simulink model "penduloDobleVersionFinal"  (R2021a)
settings: Solver=ode4  StartTime=0.0  StopTime=25  FixedStep=1e-3  RelTol=1e-3
PreLoadFcn:
  | cuentas_pendulo_doble_final;
InitFcn:
  | cuentas_pendulo_doble_final;
values from neighbouring files (symbols this model uses):
  I0 = 0    [TPF_Control_Automatico.m]    (also in cuentas_pendulo_doble_final.m)
  I1 = m1_value*(((L1_value)^2)/12)    (= 0.0833333333333)    [TPF_Control_Automatico.m]    (also in cuentas_pendulo_doble_final.m; cuentas_prueba.m = 0.0104166666667)
  I2 = m2_value*(((L2_value)^2)/12)    (= 0.1875)    [TPF_Control_Automatico.m]    (also in cuentas_pendulo_doble_final.m; cuentas_prueba.m = 0.03515625)
  K = place(sys.A, sys.B, [-3 -2.5 -2.4 -2 -1.9 -1.8])    [TPF_Control_Automatico.m]    (also in cuentas_pendulo_doble.m = acker(A,B,[0.002,-0.001,-0.001,-0.001,-0.001,-0.001]); cuentas_pendulo_doble_final.m = place(sys.A, sys.B, [-4 -3.5 -3 -2.5 -2 -1.5]); cuentas_prueba.m = acker(sys.A, sys.B, [-3 -3 -2 -2]))
  Ka = Ka(1:6)    [cuentas_pendulo_doble_final.m]    (also in cuentas_prueba.m = Ka(1:4))
  KaDisc = KDisc2(1:6)    [cuentas_pendulo_doble_final.m]    (also in cuentas_prueba.m = KDisc2(1:4))
  Kai = Ka(7)    [cuentas_pendulo_doble_final.m]    (also in cuentas_prueba.m = Ka(5))
  KaiDisc = KDisc2(7)    [cuentas_pendulo_doble_final.m]    (also in cuentas_prueba.m = KDisc2(5))
  KDisc = place(sysDisc.A, sysDisc.B, exp([-1.5 -1.6 -1.7 -2 -2.1 -2.2].*Ts))    [TPF_Control_Automatico.m]    (also in cuentas_pendulo_doble_final.m = place(sysDisc.A, sysDisc.B, exp([-3.5 -3 -2.5 -2 -1.5 -1].*T; cuentas_prueba.m = acker(sysDisc.A, sysDisc.B, exp([-2 -2 -1 -1].*Ts)))
  L = place((sys.A)',(sys.C)', [-3 -2.5 -2.4 -2 -1.9 -1.8].*10)'    [TPF_Control_Automatico.m]    (also in cuentas_pendulo_doble.m = [zeros(3,1); cuentas_pendulo_doble_final.m = place((sys.A)',(sys.C)', [-4 -3.5 -3 -2.5 -2 -1.5].*15)'; cuentas_prueba.m = place((sys.A)',(sys.C)', [-25 -20 -35 -30])')
  L1_value = 1    [TPF_Control_Automatico.m]    (also in cuentas_pendulo_doble.m = 0.5; cuentas_pendulo_doble_final.m; cuentas_prueba.m = 0.5)
  L2_value = 1.5    [TPF_Control_Automatico.m]    (also in cuentas_pendulo_doble.m = 0.75; cuentas_pendulo_doble_final.m; cuentas_prueba.m = 0.75)
  LDisc = place((sysDisc.A)',(sysDisc.C)', exp(([-1.5 -1.6 -1.7 -2 -2.1 -2.2].*20).*Ts))'    [TPF_Control_Automatico.m]    (also in cuentas_pendulo_doble_final.m = place((sysDisc.A)',(sysDisc.C)', exp(([-3.5 -3 -2.5 -2 -1.5 ; cuentas_prueba.m = place((sysDisc.A)',(sysDisc.C)', exp([-20 -15 -25 -30].*Ts)))
  m0_value = 5    [TPF_Control_Automatico.m]    (also in cuentas_pendulo_doble.m = 1.5; cuentas_pendulo_doble_final.m; cuentas_prueba.m = 1.5)
  m1_value = 1    [TPF_Control_Automatico.m]    (also in cuentas_pendulo_doble.m = 0.5; cuentas_pendulo_doble_final.m; cuentas_prueba.m = 0.5)
  m2_value = 1    [TPF_Control_Automatico.m]    (also in cuentas_pendulo_doble.m = 0.75; cuentas_pendulo_doble_final.m; cuentas_prueba.m = 0.75)
  s = tf('s')    [TPF_Control_Automatico.m]    (also in cuentas_pendulo_doble.m; cuentas_pendulo_doble_final.m; cuentas_prueba.m)
  sys = ss(A,B,C,D)    [TPF_Control_Automatico.m]    (also in cuentas_pendulo_doble_final.m; cuentas_prueba.m)
  sysDisc = c2d(sys, Ts, 'tustin')    [TPF_Control_Automatico.m]    (also in cuentas_pendulo_doble_final.m; cuentas_prueba.m)
  Ts = 0.03    [TPF_Control_Automatico.m]    (also in cuentas_pendulo_doble_final.m = 0.025; cuentas_prueba.m = 0.1)
  Ts2 = 0.01    [cuentas_pendulo_doble_final.m]    (also in cuentas_prueba.m = 0.05)
undefined symbols (not defined in the file or in its folder): DiscIntNeverNeededParam, X, Y, Z
libraries: sm_lib x100, nesl_utility x40, eeGeneralControl x5
(part 4 of 4)

== system penduloDobleVersionFinal/Control por realimentacion con obs discreto/Planta/Base ==
  Base : sm_lib/Body Elements/Brick Solid  GraphicAmbientColor=[0.15 0.15 0.15 1.0]  BasedOnType=Mass  BrickDimensions=[20 1 0.01]  BrickDimensionUnits=m  CenterOfMass=[0 0 0]  CenterOfMassUnits=m  GraphicDiffuseColor=[0.7 0.7 0.7]  Density=1000  DensityUnits=kg/m^3  DoExposeReferenceFrame=on  GraphicEmissiveColor=[0.0 0.0 0.0 1.0]  ExportEntireGeometry=off  SerializedFrames=<Frames/>  MarkerShape=Sphere  MarkerSize=10  GraphicType=FromGeometry  InertiaType=CalculateFromGeometry  Mass=10  MassUnits=kg  MomentsOfInertia=[1 1 1]  MomentsOfInertiaUnits=kg*m^2  GraphicOpacity=1.0  ProductsOfInertia=[0 0 0]  ProductsOfInertiaUnits=kg*m^2  GraphicShininess=75  GraphicSpecularColor=[0.5 0.5 0.5 1.0]  GraphicVisPropType=SimpleVisualProperties
  Base1 : sm_lib/Body Elements/Brick Solid  GraphicAmbientColor=[0.15 0.15 0.15 1.0]  BasedOnType=Mass  BrickDimensions=[20 0.05 0.0805]  BrickDimensionUnits=m  CenterOfMass=[0 0 0]  CenterOfMassUnits=m  GraphicDiffuseColor=[0.6 0.6 0.6]  Density=1000  DensityUnits=kg/m^3  DoExposeReferenceFrame=off  GraphicEmissiveColor=[0.0 0.0 0.0 1.0]  ExportEntireGeometry=off  SerializedFrames=<Frames><Frame><Id>Frame1</Id><Value><Name>F1</Name><Origin><Source>GeometricFeature</Source><FeatureName>-y +z curve</FeatureName></Origin><PrimaryAxis><DefinedDirection>+Z</DefinedDirection><Source>ReferenceFrame</Source><SourceDirection>+Z</SourceDirection><FeatureName></FeatureName></PrimaryAxis><SecondaryAxis><DefinedDirection>+X</DefinedDirection><Source>ReferenceFrame</Source><SourceDirection>+X</SourceDirection><FeatureName></FeatureName></SecondaryAxis></Value></Frame></Frames>  MarkerShape=Sphere  MarkerSize=10  GraphicType=FromGeometry  InertiaType=CalculateFromGeometry  Mass=10  MassUnits=kg  MomentsOfInertia=[1 1 1]  MomentsOfInertiaUnits=kg*m^2  GraphicOpacity=1.0  ProductsOfInertia=[0 0 0]  ProductsOfInertiaUnits=kg*m^2  GraphicShininess=75  GraphicSpecularColor=[0.5 0.5 0.5 1.0]  GraphicVisPropType=SimpleVisualProperties
  Base2 : sm_lib/Body Elements/Brick Solid  GraphicAmbientColor=[0.15 0.15 0.15 1.0]  BasedOnType=Mass  BrickDimensions=[20 0.05 0.0805]  BrickDimensionUnits=m  CenterOfMass=[0 0 0]  CenterOfMassUnits=m  GraphicDiffuseColor=[0.6 0.6 0.6]  Density=1000  DensityUnits=kg/m^3  DoExposeReferenceFrame=off  GraphicEmissiveColor=[0.0 0.0 0.0 1.0]  ExportEntireGeometry=off  SerializedFrames=<Frames><Frame><Id>Frame1</Id><Value><Name>F1</Name><Origin><Source>GeometricFeature</Source><FeatureName>-y +z curve</FeatureName></Origin><PrimaryAxis><DefinedDirection>+Z</DefinedDirection><Source>ReferenceFrame</Source><SourceDirection>+Z</SourceDirection><FeatureName></FeatureName></PrimaryAxis><SecondaryAxis><DefinedDirection>+X</DefinedDirection><Source>ReferenceFrame</Source><SourceDirection>+X</SourceDirection><FeatureName></FeatureName></SecondaryAxis></Value></Frame></Frames>  MarkerShape=Sphere  MarkerSize=10  GraphicType=FromGeometry  InertiaType=CalculateFromGeometry  Mass=10  MassUnits=kg  MomentsOfInertia=[1 1 1]  MomentsOfInertiaUnits=kg*m^2  GraphicOpacity=1.0  ProductsOfInertia=[0 0 0]  ProductsOfInertiaUnits=kg*m^2  GraphicShininess=75  GraphicSpecularColor=[0.5 0.5 0.5 1.0]  GraphicVisPropType=SimpleVisualProperties
  T1 : sm_lib/Frames and Transforms/Rigid Transform  TranslationMethod=StandardAxis  TranslationStandardOffset=-0.0255  TranslationLengthUnit=m  TranslationStandardAxis=+Z  TranslationCartesianOffset=[0 0 0]  TranslationROffset=0  TranslationROffsetUnits=m  TranslationZOffset=0  TranslationZOffsetUnits=m  TranslationThetaOffset=0  TranslationThetaOffsetUnits=deg  RotationMethod=RotationSequence  RotationAngleUnits=deg  RotationStandardAxis=+Z  RotationAngle=0.0  RotationArbitraryAxis=[0 0 1]  FollAlignAxisA=+X  BaseAlignAxisA=+Y  FollAlignAxisB=+Y  BaseAlignAxisB=+Z  RotationSequenceAxes=FollowerAxes  RotationSequence=XYZ  RotationSequenceAngles=[0 0 0]  RotationSequenceAnglesUnits=deg  RotationMatrix=[1 0 0; 0 1 0; 0 0 1]
  T2 : sm_lib/Frames and Transforms/Rigid Transform  TranslationMethod=StandardAxis  TranslationStandardOffset=0.05  TranslationLengthUnit=m  TranslationStandardAxis=+Z  TranslationCartesianOffset=[0 0 0]  TranslationROffset=0  TranslationROffsetUnits=m  TranslationZOffset=0  TranslationZOffsetUnits=m  TranslationThetaOffset=0  TranslationThetaOffsetUnits=deg  RotationMethod=RotationSequence  RotationAngleUnits=deg  RotationStandardAxis=+Z  RotationAngle=0.0  RotationArbitraryAxis=[0 0 1]  FollAlignAxisA=+X  BaseAlignAxisA=+Y  FollAlignAxisB=+Y  BaseAlignAxisB=+Z  RotationSequenceAxes=FollowerAxes  RotationSequence=XYZ  RotationSequenceAngles=[0 0 0]  RotationSequenceAnglesUnits=deg  RotationMatrix=[1 0 0; 0 1 0; 0 0 1]
  T3 : sm_lib/Frames and Transforms/Rigid Transform  TranslationMethod=StandardAxis  TranslationStandardOffset=0.5  TranslationLengthUnit=m  TranslationStandardAxis=+Y  TranslationCartesianOffset=[0 0 0]  TranslationROffset=0  TranslationROffsetUnits=m  TranslationZOffset=0  TranslationZOffsetUnits=m  TranslationThetaOffset=0  TranslationThetaOffsetUnits=deg  RotationMethod=RotationSequence  RotationAngleUnits=deg  RotationStandardAxis=+Z  RotationAngle=0.0  RotationArbitraryAxis=[0 0 1]  FollAlignAxisA=+X  BaseAlignAxisA=+Y  FollAlignAxisB=+Y  BaseAlignAxisB=+Z  RotationSequenceAxes=FollowerAxes  RotationSequence=XYZ  RotationSequenceAngles=[0 0 0]  RotationSequenceAnglesUnits=deg  RotationMatrix=[1 0 0; 0 1 0; 0 0 1]
  T4 : sm_lib/Frames and Transforms/Rigid Transform  TranslationMethod=StandardAxis  TranslationStandardOffset=0.05  TranslationLengthUnit=m  TranslationStandardAxis=+Z  TranslationCartesianOffset=[0 0 0]  TranslationROffset=0  TranslationROffsetUnits=m  TranslationZOffset=0  TranslationZOffsetUnits=m  TranslationThetaOffset=0  TranslationThetaOffsetUnits=deg  RotationMethod=RotationSequence  RotationAngleUnits=deg  RotationStandardAxis=+Z  RotationAngle=0.0  RotationArbitraryAxis=[0 0 1]  FollAlignAxisA=+X  BaseAlignAxisA=+Y  FollAlignAxisB=+Y  BaseAlignAxisB=+Z  RotationSequenceAxes=FollowerAxes  RotationSequence=XYZ  RotationSequenceAngles=[0 0 0]  RotationSequenceAnglesUnits=deg  RotationMatrix=[1 0 0; 0 1 0; 0 0 1]
  T5 : sm_lib/Frames and Transforms/Rigid Transform  TranslationMethod=StandardAxis  TranslationStandardOffset=0.55  TranslationLengthUnit=m  TranslationStandardAxis=-Y  TranslationCartesianOffset=[0 0 0]  TranslationROffset=0  TranslationROffsetUnits=m  TranslationZOffset=0  TranslationZOffsetUnits=m  TranslationThetaOffset=0  TranslationThetaOffsetUnits=deg  RotationMethod=RotationSequence  RotationAngleUnits=deg  RotationStandardAxis=+Z  RotationAngle=0.0  RotationArbitraryAxis=[0 0 1]  FollAlignAxisA=+X  BaseAlignAxisA=+Y  FollAlignAxisB=+Y  BaseAlignAxisB=+Z  RotationSequenceAxes=FollowerAxes  RotationSequence=XYZ  RotationSequenceAngles=[0 0 0]  RotationSequenceAnglesUnits=deg  RotationMatrix=[1 0 0; 0 1 0; 0 0 1]
  Conn2 : PMIOPort  Side=Right
  Conn1 : PMIOPort  Port=2  Side=Right
  Conn3 : PMIOPort  Port=3  Side=Right
  connections:
  Base/RConn1 -- T1/RConn1
  Base1/LConn1 -- T3/RConn1
  T1/LConn1 -- Conn1/RConn1
  T2/LConn1 -- Conn2/RConn1
  T3/LConn1 -- T2/RConn1
  T5/LConn1 -- T4/RConn1
  Base2/LConn1 -- T5/RConn1
  T4/LConn1 -- Conn3/RConn1
